simulink model "PC_Quadcopter_Simulation_DoB_ADRC_Hexacopter"  (R2021a)
settings: Solver=ode4  StartTime=0.0  StopTime=30  FixedStep=0.01  MaxStep=0.06  RelTol=1e-3
PreLoadFcn:
  | DoB_parameter
model workspace (MAT data in the model file):
  Sig : Simulink.Signal (value not decoded)
values from neighbouring files (symbols this model uses):
  A = [ ... (first row only)    [DoB_parameter.m]
  B = [0 1 0]'    [DoB_parameter.m]
  C = [1 0 0]    [DoB_parameter.m]
  den_Inv_X = conv(num_X,den_Qfilter)    [DoB_parameter.m]
  den_Inv_Y = conv(num_Y, den_Qfilter)    [DoB_parameter.m]
  den_Inv_Z = conv(num_Z, den_Qfilter_Z)    [DoB_parameter.m]
  den_Qfilter = [1 a1/tau a0/tau^2]    [DoB_parameter.m]
  den_Qfilter_Z = [1 a1/tau a0/tau^2]    [DoB_parameter.m]
  I_xx = J(1,1)    [DoB_parameter.m]
  I_yy = J(2,2)    [DoB_parameter.m]
  I_zz = J(3,3)    [DoB_parameter.m]
  IC = block.DialogPrm(2).Data    [quadcopterDynamicsSFunction.m]
  L = [l1 l2 l3]'    [DoB_parameter.m]
  num_Inv_X = conv(den_X,num_Qfilter)    [DoB_parameter.m]
  num_Inv_Y = conv(den_Y, num_Qfilter)    [DoB_parameter.m]
  num_Inv_Z = conv(den_Z, num_Qfilter_Z)    [DoB_parameter.m]
  num_Qfilter = a0/tau^2    (= 100)    [DoB_parameter.m]
  num_Qfilter_Z = a0/tau^2    (= 11.1111111111)    [DoB_parameter.m]
undefined symbols (not defined in the file or in its folder): magnitude, quadModel
libraries: simulink x13, sharedTrackingLibrary x1
(part 2 of 2)

== system PC_Quadcopter_Simulation_DoB_ADRC_Hexacopter/LESO/Linear Extended-State Observer ==
  y : Inport
  u : Inport  Port=2
  Add3 : Sum  Inputs=+++
  Demux : Demux  Outputs=3
  Integrator : Integrator
  Terminator : Terminator
  theta1 : Gain  Gain=B  Multiplication=Matrix(K*u)
  theta10 : Gain  Gain=L  Multiplication=Matrix(K*u)
  theta2 : Gain  Gain=A-L*C  Multiplication=Matrix(K*u)
  x2_hat : Outport
  x3_hat (F) : Outport  Port=2
  wires:
  theta1/1 -> Add3/2
  theta10/1 -> Add3/1
  y/1 -> theta10/1
  u/1 -> theta1/1
  Add3/1 -> Integrator/1
  theta2/1 -> Add3/3
  Demux/3 -> x3_hat (F)/1
  Demux/2 -> x2_hat/1
  Integrator/1 -> theta2/1, Demux/1
  Demux/1 -> Terminator/1

== system PC_Quadcopter_Simulation_DoB_ADRC_Hexacopter/LESO/Linear Extended-State Observer1 ==
  y : Inport
  u : Inport  Port=2
  Add3 : Sum  Commented=on  Inputs=+++
  Demux : Demux  Commented=on  Outputs=3
  Integrator : Integrator  Commented=on
  Terminator : Terminator  Commented=on
  theta1 : Gain  Commented=on  Gain=B  Multiplication=Matrix(K*u)
  theta10 : Gain  Commented=on  Gain=L  Multiplication=Matrix(K*u)
  theta2 : Gain  Commented=on  Gain=A-L*C  Multiplication=Matrix(K*u)
  x2_hat : Outport
  x3_hat (F) : Outport  Port=2
  wires:
  Demux/1 -> Terminator/1
  Integrator/1 -> Demux/1, theta2/1
  Demux/2 -> x2_hat/1
  Demux/3 -> x3_hat (F)/1
  theta2/1 -> Add3/3
  Add3/1 -> Integrator/1
  u/1 -> theta1/1
  y/1 -> theta10/1
  theta10/1 -> Add3/1
  theta1/1 -> Add3/2

== system PC_Quadcopter_Simulation_DoB_ADRC_Hexacopter/LESO/Linear Extended-State Observer2 ==
  y : Inport
  u : Inport  Port=2
  Add3 : Sum  Inputs=+++
  Demux : Demux  Outputs=3
  Integrator : Integrator
  Terminator : Terminator
  theta1 : Gain  Gain=B  Multiplication=Matrix(K*u)
  theta10 : Gain  Gain=L  Multiplication=Matrix(K*u)
  theta2 : Gain  Gain=A-L*C  Multiplication=Matrix(K*u)
  x2_hat : Outport
  x3_hat (F) : Outport  Port=2
  wires:
  theta1/1 -> Add3/2
  theta10/1 -> Add3/1
  y/1 -> theta10/1
  u/1 -> theta1/1
  Add3/1 -> Integrator/1
  theta2/1 -> Add3/3
  Demux/3 -> x3_hat (F)/1
  Demux/2 -> x2_hat/1
  Integrator/1 -> theta2/1, Demux/1
  Demux/1 -> Terminator/1

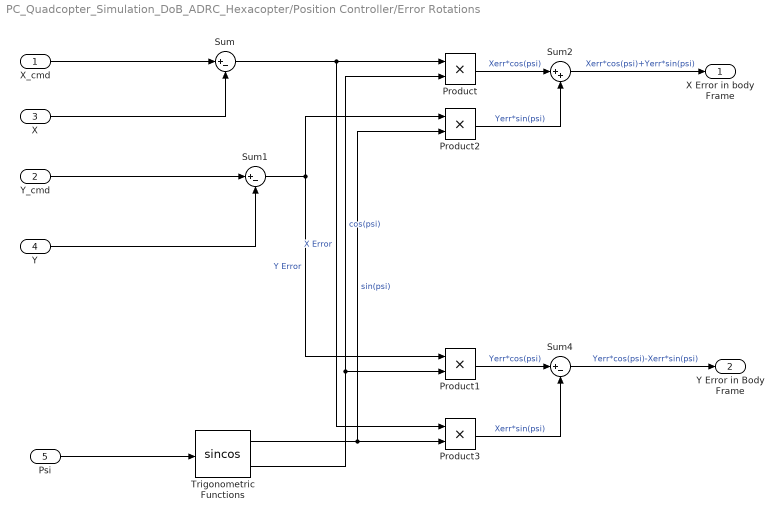
== system PC_Quadcopter_Simulation_DoB_ADRC_Hexacopter/Position Controller/Error Rotations ==
  X_cmd : Inport
  Y_cmd : Inport  Port=2
  X : Inport  Port=3
  Y : Inport  Port=4
  Psi : Inport  Port=5
  Product{,1..3} (4 alike) : Product
  Sum : Sum  Inputs=|+-
  Sum1 : Sum  Inputs=|+-
  Sum2 : Sum  Inputs=|++
  Sum4 : Sum  Inputs=|+-
  Trigonometric Functions : Trigonometry  Operator=sincos
  X Error in body Frame : Outport
  Y Error in Body Frame : Outport  Port=2
  wires:
  Sum4/1 -> Y Error in Body Frame/1  "Yerr*cos(psi)-Xerr*sin(psi)"
  Product3/1 -> Sum4/2  "Xerr*sin(psi)"
  Sum1/1 -> Product2/1, Product1/1  "Y Error"
  Trigonometric Functions/1 -> Product2/2, Product3/2  "sin(psi)"
  Sum2/1 -> X Error in body Frame/1  "Xerr*cos(psi)+Yerr*sin(psi)"
  Y_cmd/1 -> Sum1/1
  X_cmd/1 -> Sum/1
  X/1 -> Sum/2
  Y/1 -> Sum1/2
  Sum/1 -> Product3/1, Product/1  "X Error"
  Trigonometric Functions/2 -> Product/2, Product1/2  "cos(psi)"
  Product/1 -> Sum2/1  "Xerr*cos(psi)"
  Product2/1 -> Sum2/2  "Yerr*sin(psi)"
  Product1/1 -> Sum4/1  "Yerr*cos(psi)"
  Psi/1 -> Trigonometric Functions/1

== system PC_Quadcopter_Simulation_DoB_ADRC_Hexacopter/Position Controller/Phi Command Control ==
  note: -1 Gain is required because a "negative"
      | angle of Phi induces a positive velocity
      | in the body frame y direction!
  Desired Yb Velocity : Inport
  Yb Velocity : Inport  Port=2
  Attitude Limits_Phi : Saturate  UpperLimit=ASat  LowerLimit=-ASat
  Gain : Gain  Gain=-1
  Kdp : Gain  Gain=Kd
  Kpp : Gain  Gain=Kp
  Sum3 : Sum  Inputs=|+-
  Sum6 : Sum  Inputs=|+-
  V Derivative : Derivative
  Phi_cmd : Outport
  wires:
  V Derivative/1 -> Kdp/1
  Attitude Limits_Phi/1 -> Phi_cmd/1  "Phi_cmd"
  Sum6/1 -> Gain/1
  Kpp/1 -> Sum6/1
  Sum3/1 -> Kpp/1  "Velocity Error"
  Yb Velocity/1 -> V Derivative/1, Sum3/2
  Desired Yb Velocity/1 -> Sum3/1
  Gain/1 -> Attitude Limits_Phi/1
  Kdp/1 -> Sum6/2

== system PC_Quadcopter_Simulation_DoB_ADRC_Hexacopter/Position Controller/Theta Command Control ==
  Desired Xb Velocity : Inport
  Xb Velocity : Inport  Port=2
  Attitude Limits_Theta : Saturate  UpperLimit=ASat  LowerLimit=-ASat
  Kdt : Gain  Gain=Kd
  Kpt : Gain  Gain=Kp
  Sum3 : Sum  Inputs=|+-
  Sum6 : Sum  Inputs=|+-
  U Derivative : Derivative
  The_cmd : Outport
  wires:
  Kdt/1 -> Sum6/2
  U Derivative/1 -> Kdt/1
  Attitude Limits_Theta/1 -> The_cmd/1  "The_cmd"
  Sum6/1 -> Attitude Limits_Theta/1
  Kpt/1 -> Sum6/1
  Sum3/1 -> Kpt/1  "Velocity Error"
  Xb Velocity/1 -> U Derivative/1, Sum3/2
  Desired Xb Velocity/1 -> Sum3/1

== system PC_Quadcopter_Simulation_DoB_ADRC_Hexacopter/Hexacopter Dynamics/Motor Dynamics/Throttle To RPM Gain and Cutoff_1 ==
  note: minThr should be a quad.mat value
  note: This gain should be a quad.mat value
  note: This constant should be a quad.mat value
  note: Output equals linearly scaled RPM
      | for given throttle input if throttle input >=Throttle Cuttoff (minThr)
      | else output is zero.
  In5 : Inport
  Constant : Constant  Value=quadModel.b
  Gain : Gain  Gain=quadModel.cr
  Minimum Throttle Cutoff : simulink/Logic and Bit Operations/Compare To Constant  relop=>=  const=quadModel.minThr  OutDataTypeStr=uint8
  Product : Product
  Sum1 : Sum  Inputs=++|
  Out5 : Outport
  wires:
  Minimum Throttle Cutoff/1 -> Product/2
  Product/1 -> Out5/1
  In5/1 -> Gain/1, Minimum Throttle Cutoff/1
  Gain/1 -> Sum1/2
  Sum1/1 -> Product/1
  Constant/1 -> Sum1/1

== system PC_Quadcopter_Simulation_DoB_ADRC_Hexacopter/Hexacopter Dynamics/Motor Dynamics/Throttle To RPM Gain and Cutoff_2 ==
  note: minThr should be a quad.mat value
  note: This gain should be a quad.mat value
  note: This constant should be a quad.mat value
  note: Output equals linearly scaled RPM
      | for given throttle input if throttle input >=Throttle Cuttoff (minThr)
      | else output is zero.
  In5 : Inport
  Constant : Constant  Value=quadModel.b
  Gain : Gain  Gain=quadModel.cr
  Minimum Throttle Cutoff : simulink/Logic and Bit Operations/Compare To Constant  relop=>=  const=quadModel.minThr  OutDataTypeStr=uint8
  Product : Product
  Sum1 : Sum  Inputs=++|
  Out5 : Outport
  wires:
  Minimum Throttle Cutoff/1 -> Product/2
  Product/1 -> Out5/1
  In5/1 -> Gain/1, Minimum Throttle Cutoff/1
  Gain/1 -> Sum1/2
  Sum1/1 -> Product/1
  Constant/1 -> Sum1/1

== system PC_Quadcopter_Simulation_DoB_ADRC_Hexacopter/Hexacopter Dynamics/Motor Dynamics/Throttle To RPM Gain and Cutoff_3 ==
  note: minThr should be a quad.mat value
  note: This gain should be a quad.mat value
  note: This constant should be a quad.mat value
  note: Output equals linearly scaled RPM
      | for given throttle input if throttle input >=Throttle Cuttoff (minThr)
      | else output is zero.
  In5 : Inport
  Constant : Constant  Value=quadModel.b
  Gain : Gain  Gain=quadModel.cr
  Minimum Throttle Cutoff : simulink/Logic and Bit Operations/Compare To Constant  relop=>=  const=quadModel.minThr  OutDataTypeStr=uint8
  Product : Product
  Sum1 : Sum  Inputs=++|
  Out5 : Outport
  wires:
  Minimum Throttle Cutoff/1 -> Product/2
  Product/1 -> Out5/1
  In5/1 -> Gain/1, Minimum Throttle Cutoff/1
  Gain/1 -> Sum1/2
  Sum1/1 -> Product/1
  Constant/1 -> Sum1/1

== system PC_Quadcopter_Simulation_DoB_ADRC_Hexacopter/Hexacopter Dynamics/Motor Dynamics/Throttle To RPM Gain and Cutoff_4 ==
  note: minThr should be a quad.mat value
  note: This gain should be a quad.mat value
  note: This constant should be a quad.mat value
  note: Output equals linearly scaled RPM
      | for given throttle input if throttle input >=Throttle Cuttoff (minThr)
      | else output is zero.
  In5 : Inport
  Constant : Constant  Value=quadModel.b
  Gain : Gain  Gain=quadModel.cr
  Minimum Throttle Cutoff : simulink/Logic and Bit Operations/Compare To Constant  relop=>=  const=quadModel.minThr  OutDataTypeStr=uint8
  Product : Product
  Sum1 : Sum  Inputs=++|
  Out5 : Outport
  wires:
  Minimum Throttle Cutoff/1 -> Product/2
  Product/1 -> Out5/1
  In5/1 -> Gain/1, Minimum Throttle Cutoff/1
  Gain/1 -> Sum1/2
  Sum1/1 -> Product/1
  Constant/1 -> Sum1/1

== system PC_Quadcopter_Simulation_DoB_ADRC_Hexacopter/Hexacopter Dynamics/Motor Dynamics/Throttle To RPM Gain and Cutoff_5 ==
  note: minThr should be a quad.mat value
  note: This gain should be a quad.mat value
  note: This constant should be a quad.mat value
  note: Output equals linearly scaled RPM
      | for given throttle input if throttle input >=Throttle Cuttoff (minThr)
      | else output is zero.
  In5 : Inport
  Constant : Constant  Value=quadModel.b
  Gain : Gain  Gain=quadModel.cr
  Minimum Throttle Cutoff : simulink/Logic and Bit Operations/Compare To Constant  relop=>=  const=quadModel.minThr  OutDataTypeStr=uint8
  Product : Product
  Sum1 : Sum  Inputs=++|
  Out5 : Outport
  wires:
  Minimum Throttle Cutoff/1 -> Product/2
  Product/1 -> Out5/1
  In5/1 -> Gain/1, Minimum Throttle Cutoff/1
  Gain/1 -> Sum1/2
  Sum1/1 -> Product/1
  Constant/1 -> Sum1/1

== system PC_Quadcopter_Simulation_DoB_ADRC_Hexacopter/Hexacopter Dynamics/Motor Dynamics/Throttle To RPM Gain and Cutoff_6 ==
  note: minThr should be a quad.mat value
  note: This gain should be a quad.mat value
  note: This constant should be a quad.mat value
  note: Output equals linearly scaled RPM
      | for given throttle input if throttle input >=Throttle Cuttoff (minThr)
      | else output is zero.
  In5 : Inport
  Constant : Constant  Value=quadModel.b
  Gain : Gain  Gain=quadModel.cr
  Minimum Throttle Cutoff : simulink/Logic and Bit Operations/Compare To Constant  relop=>=  const=quadModel.minThr  OutDataTypeStr=uint8
  Product : Product
  Sum1 : Sum  Inputs=++|
  Out5 : Outport
  wires:
  Minimum Throttle Cutoff/1 -> Product/2
  Product/1 -> Out5/1
  In5/1 -> Gain/1, Minimum Throttle Cutoff/1
  Gain/1 -> Sum1/2
  Sum1/1 -> Product/1
  Constant/1 -> Sum1/1

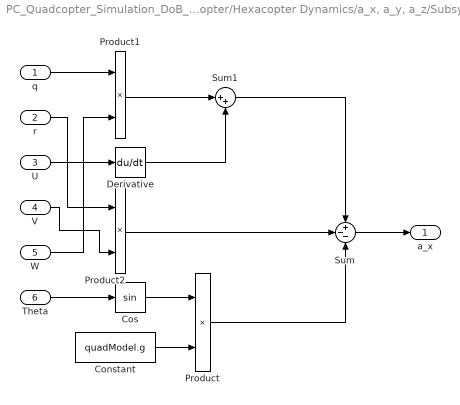
== system PC_Quadcopter_Simulation_DoB_ADRC_Hexacopter/Hexacopter Dynamics/a_x, a_y, a_z/Subsystem ==
  q : Inport
  r : Inport  Port=2
  U : Inport  Port=3
  V : Inport  Port=4
  W : Inport  Port=5
  Theta : Inport  Port=6
  Constant : Constant  Value=quadModel.g
  Cos : Trigonometry
  Derivative : Derivative
  Product : Product
  Product1 : Product
  Product2 : Product
  Sum : Sum  Inputs=+--
  Sum1 : Sum  Inputs=|++
  a_x : Outport
  wires:
  Theta/1 -> Cos/1
  Cos/1 -> Product/1
  Constant/1 -> Product/2
  Product1/1 -> Sum1/1
  Derivative/1 -> Sum1/2
  Sum1/1 -> Sum/1
  Sum/1 -> a_x/1
  Product2/1 -> Sum/2
  Product/1 -> Sum/3
  U/1 -> Derivative/1
  q/1 -> Product1/1
  W/1 -> Product1/2
  r/1 -> Product2/1
  V/1 -> Product2/2

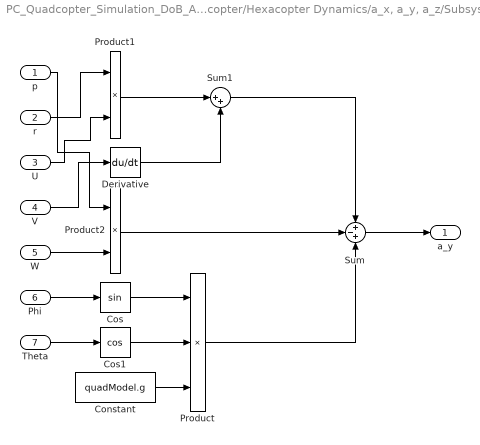
== system PC_Quadcopter_Simulation_DoB_ADRC_Hexacopter/Hexacopter Dynamics/a_x, a_y, a_z/Subsystem1 ==
  p : Inport
  r : Inport  Port=2
  U : Inport  Port=3
  V : Inport  Port=4
  W : Inport  Port=5
  Phi : Inport  Port=6
  Theta : Inport  Port=7
  Constant : Constant  Value=quadModel.g
  Cos : Trigonometry
  Cos1 : Trigonometry  Operator=cos
  Derivative : Derivative
  Product : Product  Inputs=3
  Product1 : Product
  Product2 : Product
  Sum : Sum  Inputs=+-+
  Sum1 : Sum  Inputs=|++
  a_y : Outport
  wires:
  V/1 -> Derivative/1
  Theta/1 -> Cos1/1
  Phi/1 -> Cos/1
  Cos/1 -> Product/1
  Cos1/1 -> Product/2
  Constant/1 -> Product/3
  Derivative/1 -> Sum1/2
  r/1 -> Product1/1
  U/1 -> Product1/2
  W/1 -> Product2/2
  p/1 -> Product2/1
  Product1/1 -> Sum1/1
  Product2/1 -> Sum/2
  Sum1/1 -> Sum/1
  Product/1 -> Sum/3
  Sum/1 -> a_y/1

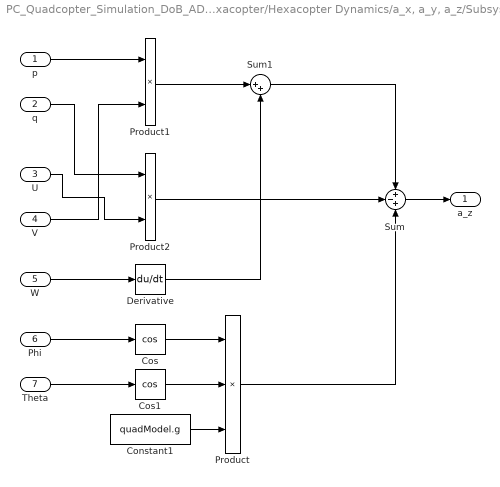
== system PC_Quadcopter_Simulation_DoB_ADRC_Hexacopter/Hexacopter Dynamics/a_x, a_y, a_z/Subsystem2 ==
  p : Inport
  q : Inport  Port=2
  U : Inport  Port=3
  V : Inport  Port=4
  W : Inport  Port=5
  Phi : Inport  Port=6
  Theta : Inport  Port=7
  Constant1 : Constant  Value=quadModel.g
  Cos : Trigonometry  Operator=cos
  Cos1 : Trigonometry  Operator=cos
  Derivative : Derivative
  Product : Product  Inputs=3
  Product1 : Product
  Product2 : Product
  Sum : Sum  Inputs=+-+
  Sum1 : Sum  Inputs=|++
  a_z : Outport
  wires:
  Cos1/1 -> Product/2
  Constant1/1 -> Product/3
  Cos/1 -> Product/1
  Sum/1 -> a_z/1
  Theta/1 -> Cos1/1
  Phi/1 -> Cos/1
  W/1 -> Derivative/1
  p/1 -> Product1/1
  V/1 -> Product1/2
  q/1 -> Product2/1
  U/1 -> Product2/2
  Product1/1 -> Sum1/1
  Derivative/1 -> Sum1/2
  Product2/1 -> Sum/2
  Sum1/1 -> Sum/1
  Product/1 -> Sum/3

== matlab function PC_Quadcopter_Simulation_DoB_ADRC_Hexacopter/Fault Diagnosis/Generate Residual/MATLAB Function - Generate Predicted Output ==
  data: xEstimated input; yPredicted output; u input
function yPredicted = generatePredictedOutput(xEstimated,u)

%   Copyright 2017 The MathWorks, Inc.

%#codegen

% Given state estimates at previous time (k-1) utilizing measurements up to
% (k-1), predict states at current step.
xPredicted = myStateTransitionFcn(xEstimated,u); % xhat[k|k-1]
% Generate output estimate, again without utilizing the measurement at
% current time.
yPredicted = myMeasurementFcn(xPredicted); % y[k|k-1]
end

== matlab function PC_Quadcopter_Simulation_DoB_ADRC_Hexacopter/Hexacopter Control Mixing/MATLAB Function ==
  data: u input; y output
function y = fcn(u)
%% mixing matrix: PID correction to motors
m = 1.023;
g = 9.81;
ct = 1.4865e-07;
cr = 80.5840;
b = 976.2;
%% health state 6*1
h = u(5:10,1);
FDI = u(11,1);
% 
% A = [
%     -1/h(1,1) -1/h(1,1) -1/h(1,1) 1/h(1,1)
%     1/h(2,1) -1/h(2,1) 1/h(2,1) 1/h(2,1)
%     1/h(3,1) 0 -1/h(3,1) 1/h(3,1)
%     1/h(4,1) 1/h(4,1) 1/h(4,1) 1/h(4,1)
%     -1/h(5,1) 1/h(5,1) -1/h(5,1) 1/h(5,1)
%     -1/h(6,1) 0 1/h(6,1) 1/h(6,1)
%     ];

A = [
    -1 -1 -1 1
    1 -1 1 1
    1 0 -1 1
    1 1 1 1
    -1 1 -1 1
    -1 0 1 1
    ];

%% 고장을 고려한 mixing 변화
if FDI==1 | FDI==4
h(1,1)=0;
h(2,1)=1;
h(3,1)=1;
h(4,1)=0;
h(5,1)=1;
h(6,1)=1;

A = [
    -1 -1 -1 1
    1 -1 1 1
    1 0 -1 1
    1 1 1 1
    -1 1 -1 1
    -1 0 1 1
    ];

elseif FDI==2 | FDI==5
h(1,1)=1;
h(2,1)=0;
h(3,1)=1;
h(4,1)=1;
h(5,1)=0;
h(6,1)=1;

A = [
    -1 -1 -1 1
    1 -1 1 1
    1 0 -1 1
    1 1 1 1
    -1 1 -1 1
    -1 0 1 1
    ];

elseif FDI==3 | FDI==6
h(1,1)=1;
h(2,1)=1;
h(3,1)=0;
h(4,1)=1;
h(5,1)=1;
h(6,1)=0;
% 
A = [
    -1 -1 -1 1
    1 -1 1 1
    1 0 -1 1
    1 1 1 1
    -1 1 -1 1
    -1 0 1 1
    ];

end
for i=1:6
    A(i,:) = h(i)*A(i,:);
end

%% 고장을 고려한 건강한 모터의 추력 증가
% A = sqrt(6/sum(h))*A;


y = A*( u(1:4,:) )
% y = A*( u(1:4,:) ) + (sqrt(m*g/sum(h)/ct)-b)/cr ...
%     - (sqrt(m*g/6/ct)-b)/cr ;

== matlab function PC_Quadcopter_Simulation_DoB_ADRC_Hexacopter/Fault Diagnosis/MATLAB Function ==
  data: p input; y output; q input; r input; a_z input; Z input; h input; t input
function y = FDI(p,q,r,a_z,Z,h,t)
% th = 0.04;
p_th = 0.03;
q_th = 0.07;
r_th = 0.015;
% z_th = 0.001;
%  & a_z<-z_th
y=0;

while y==0
    if  Z>0 & p>p_th & q>q_th & r>r_th & h(1) < 0.88 | t>0.2 & h(1) < 0.6
        y=1;
    elseif Z>0 & p<-p_th & q>q_th & r<-r_th & h(2) < 0.88 | t>0.2 & h(2) < 0.6
        y=2;
    elseif Z>0 & p<-p_th & -q_th<q & q<q_th & r>r_th & h(3) < 0.88 | t>0.2 & h(3) < 0.6
        y=3;
    elseif Z>0 & p<-p_th & q<-q_th & r<-r_th & h(4) < 0.88 | t>0.2 & h(4) < 0.6
        y=4;
    elseif Z>0 & p>p_th & q<-q_th & r>r_th & h(5) < 0.88 | t>0.2 & h(5) < 0.6
        y=5;
%     elseif Z>0 & p>p_th & -q_th<q & q<q_th & r<-r_th  & h(6) < 0.88 | t>0.2 & h(6) < 0.6
%         y=6;
    end
    break
end            
end

== matlab function PC_Quadcopter_Simulation_DoB_ADRC_Hexacopter/Fault Diagnosis/MATLAB Function1 ==
  data: R1 input; y output; R2 input; R3 input; R4 input; R5 input; R6 input; Z input; h input; t input
function y = FDI(R1,R2,R3,R4,R5,R6,Z,h,t)
% th = 0.04;
RPM_th = 1000;

y=0;

while y==0
    if  Z>0 & t>0.5 & R1>RPM_th & h(1) < 0.6 
%         | t>0.2 & h(1) < 0.55
        y=1;
    elseif Z>0 & t>0.5 & R2>RPM_th & h(2) < 0.6 
        y=2;
    elseif Z>0 & t>0.5 & R3>RPM_th & h(3) < 0.6 
%         | t>0.5 & h(3) < 0.6
        y=3;
    elseif Z>0 & t>0.5 & R4>RPM_th & h(4) < 0.6 
        y=4;
    elseif Z>0 & t>0.5 & R5>RPM_th & h(5) < 0.6 
        y=5;
%     elseif Z>0 & t>0.5 & R6>RPM_th & h(6) < 0.6 | Z>0 & t>0.5 & R6<-RPM_th & h(6) < 0.6
%         y=6;
    end
    break
end            
end
